simulink model "bsg_model"  (R2023a)
settings: Solver=VariableStepAuto  StartTime=0.0  StopTime=10.0  RelTol=1e-3
settings Model: Creator=Pedro  LastModifiedBy=Pedro

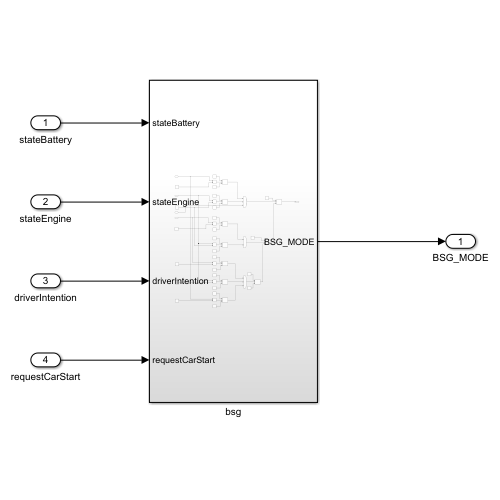
[thumbnail: Simulink's stored preview of the top-level diagram]
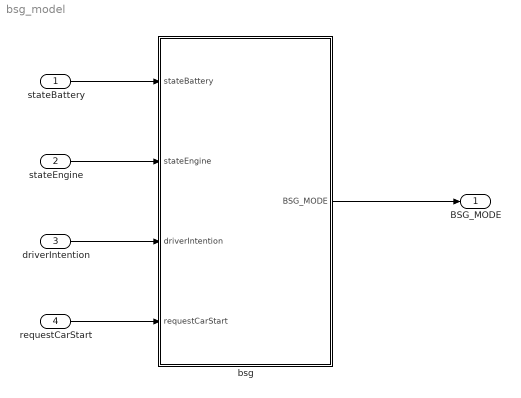
== system bsg_model ==
  stateBattery : Inport
  stateEngine : Inport  Port=2
  driverIntention : Inport  Port=3
  requestCarStart : Inport  Port=4
  bsg : Subsystem
  BSG_MODE : Outport
  wires:
  stateBattery/1 -> bsg/1(stateBattery)
  stateEngine/1 -> bsg/2(stateEngine)
  driverIntention/1 -> bsg/3(driverIntention)
  requestCarStart/1 -> bsg/4(requestCarStart)
  bsg/1(BSG_MODE) -> BSG_MODE/1

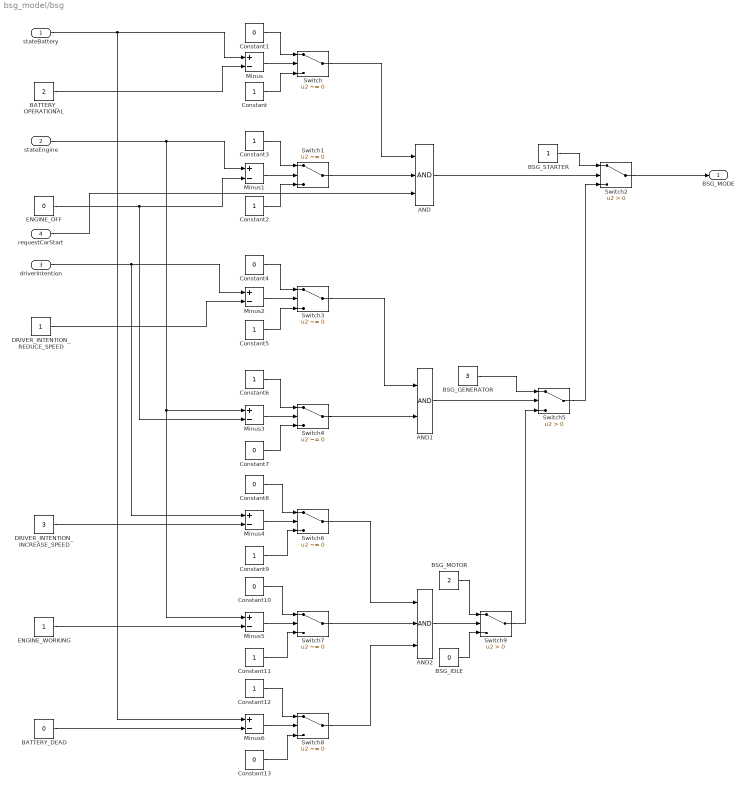
== system bsg_model/bsg ==
  stateBattery : Inport
  stateEngine : Inport  Port=2
  driverIntention : Inport  Port=3
  requestCarStart : Inport  Port=4
  AND : Logic  Inputs=3  IconShape=distinctive  AllPortsSameDT=off  OutDataTypeStr=boolean
  AND1 : Logic  IconShape=distinctive  AllPortsSameDT=off  OutDataTypeStr=boolean
  AND2 : Logic  Inputs=3  IconShape=distinctive  AllPortsSameDT=off  OutDataTypeStr=boolean
  BATTERY_DEAD : Constant  Value=0
  BATTERY_OPERATIONAL : Constant  Value=2
  BSG_GENERATOR : Constant  Value=3
  BSG_IDLE : Constant  Value=0
  BSG_MOTOR : Constant  Value=2
  BSG_STARTER : Constant
  Constant{,2..3,5..6,9,11..12} (8 alike) : Constant
  Constant{1,4,7..8,10,13} (6 alike) : Constant  Value=0
  DRIVER_INTENTION_INCREASE_SPEED : Constant  Value=3
  DRIVER_INTENTION_REDUCE_SPEED : Constant
  ENGINE_OFF : Constant  Value=0
  ENGINE_WORKING : Constant  SampleTime=-1
  Minus{,1..6} (7 alike) : Sum  Inputs=+-
  Switch{,1,3..4,6..8} (7 alike) : Switch  Criteria=u2 ~= 0  SaturateOnIntegerOverflow=off  InputSameDT=off
  Switch2 : Switch  Criteria=u2 > Threshold  SaturateOnIntegerOverflow=off  InputSameDT=off
  Switch5 : Switch  Criteria=u2 > Threshold  SaturateOnIntegerOverflow=off  InputSameDT=off
  Switch9 : Switch  Criteria=u2 > Threshold  SaturateOnIntegerOverflow=off  InputSameDT=off
  BSG_MODE : Outport
  wires:
  Constant7/1 -> Switch4/3
  Constant6/1 -> Switch4/1
  stateBattery/1 -> Minus6/1, Minus/1
  Minus5/1 -> Switch7/2
  DRIVER_INTENTION_INCREASE_SPEED/1 -> Minus4/2
  Constant4/1 -> Switch3/1
  BATTERY_OPERATIONAL/1 -> Minus/2
  Switch4/1 -> AND1/2
  stateEngine/1 -> Minus1/1, Minus3/1, Minus5/1
  Minus1/1 -> Switch1/2
  AND/1 -> Switch2/2
  AND1/1 -> Switch5/2
  Minus3/1 -> Switch4/2
  Constant2/1 -> Switch1/3
  BSG_IDLE/1 -> Switch9/3
  ENGINE_OFF/1 -> Minus3/2, Minus1/2
  Constant3/1 -> Switch1/1
  Constant8/1 -> Switch6/1
  Constant9/1 -> Switch6/3
  BATTERY_DEAD/1 -> Minus6/2
  ENGINE_WORKING/1 -> Minus5/2
  Minus/1 -> Switch/2
  Switch8/1 -> AND2/3
  Constant5/1 -> Switch3/3
  Constant10/1 -> Switch7/1
  Switch1/1 -> AND/2
  Minus2/1 -> Switch3/2
  Switch2/1 -> BSG_MODE/1
  Minus6/1 -> Switch8/2
  Constant12/1 -> Switch8/1
  BSG_STARTER/1 -> Switch2/1
  DRIVER_INTENTION_REDUCE_SPEED/1 -> Minus2/2
  Switch6/1 -> AND2/1
  Constant13/1 -> Switch8/3
  Switch7/1 -> AND2/2
  Switch3/1 -> AND1/1
  BSG_GENERATOR/1 -> Switch5/1
  Minus4/1 -> Switch6/2
  AND2/1 -> Switch9/2
  Switch5/1 -> Switch2/3
  driverIntention/1 -> Minus4/1, Minus2/1
  Constant11/1 -> Switch7/3
  Switch/1 -> AND/1
  Switch9/1 -> Switch5/3
  requestCarStart/1 -> AND/3
  Constant/1 -> Switch/3
  BSG_MOTOR/1 -> Switch9/1
  Constant1/1 -> Switch/1
